simulink library "pelib"  (R2021a)
settings: Solver=VariableStepAuto  StartTime=0.0  StopTime=10.0  RelTol=1e-3
libraries: hdlBasic x7
settings Model: Creator=asc8  LastModifiedBy=asc8

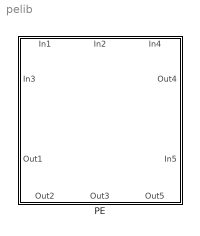
== system pelib ==
  PE : Subsystem
      settings: PortSchema="{\"entries\":[{\"content\":{\"sides\":[{\"content\":{\"connectorIds\":[\"In1\",\"Out5\"]},\"type\":\"ConnectorPlacement.EquallySpacedRectSide\",\"uuid\":\"f7e55443-70fb-4ed5-ab4f-147f7311106a\"},{\"content\":{\"connectorIds\":[\"Out1\",\"In5\"],\"side\":\"RIGHT\"},\"type\":\"ConnectorPlacement.EquallySpacedRectSide\",\"uuid\":\"6de0769a-4a22-4abb-b630-26d0c175204f\"},{\"content\":{\"connectorIds\":[\"In2\",\"In3\",\"In4\"],\"side\":\"TOP\"},\"type\":\"ConnectorPlacement.EquallySpacedRectSide\",\"uuid\":\"a041cc58-78e8-4444-b053-dd6f2c27badd\"},{\"content\":{\"connectorIds\":[\"Out2\",\"Out3\",\"Out4\"],\"side\":\"BOTTOM\"},\"type\":\"ConnectorPlacement.EquallySpacedRectSide\",\"uuid\":\"085ff6f5-8624-4aab-b622-9beedcd77ebd\"}]},\"type\":\"ConnectorPlacement.EquallySpacedConnector\",\"uuid\":\"928950cd-8b9e-4ebf-b8fd-b98c3e494fdc\"}],\"packageUris\":[\"http://schema.mathworks.com/mf0/Connector/R2020b\"],\"version\":\"1.0\"}"

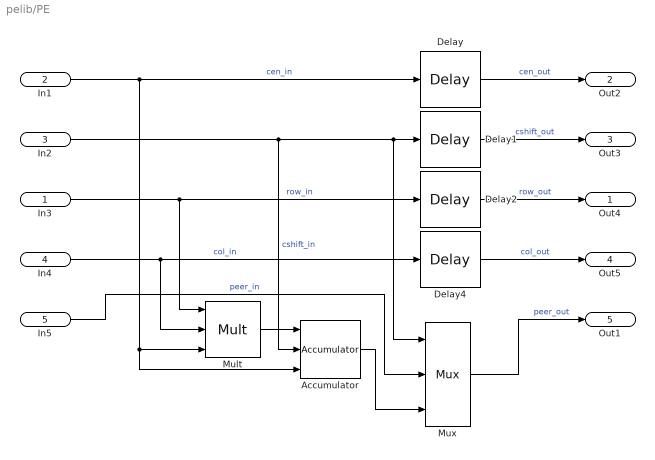
== system pelib/PE ==
  In3 : Inport
  In1 : Inport  Port=2
  In2 : Inport  Port=3
  In4 : Inport  Port=4
  In5 : Inport  Port=5
  Accumulator : hdlBasic/Accumulator  operation=Add  n_bits=16  overflow=Wrap  scale=1  rst=on  hasbypass=on  en=on  latency=1  msb_inp=100  msb=100  lsb=-100  use_behavioral_HDL=on  implementation=Fabric  XmcBlockStatus=1  maskContainerNames=group3  block_type=accum  block_config=sysgen:Accum_config
  Delay{,1..2,4} (4 alike) : hdlBasic/Delay  rst=off  en=off  latency=1  reg_retiming=off  XmcBlockStatus=1  maskContainerNames=group1  block_type=delay  block_config=sysgen:Delay_config
  Mult : hdlBasic/Mult  precision=User Defined  arith_type="Signed  (2's comp)"  n_bits=16  bin_pt=0  quantization=Truncate  overflow=Wrap  en=on  latency=2  use_behavioral_HDL=off  opt=Speed  use_embedded=on  optimum_pipeline=off  pipeline=on  use_rpm=on  placement_style=Triangular  XmcBlockStatus=1  maskContainerNames=group1  block_type=mult  block_config=sysgen:Mult_config
  Mux : hdlBasic/Mux  inputs=2  en=off  latency=0  precision=Full  arith_type=Unsigned  n_bits=16  bin_pt=14  quantization=Truncate  overflow=Wrap  XmcBlockStatus=1  maskContainerNames=tabcontainer1  block_type=mux  block_config=sysgen:Mux_config
  Out4 : Outport
  Out2 : Outport  Port=2
  Out3 : Outport  Port=3
  Out5 : Outport  Port=4
  Out1 : Outport  Port=5
  wires:
  In3/1 -> Mult/1, Delay2/1  "row_in"
  In4/1 -> Delay4/1, Mult/2  "col_in"
  In1/1 -> Mult/3, Accumulator/3, Delay/1  "cen_in"
  In2/1 -> Accumulator/2, Delay1/1, Mux/1  "cshift_in"
  Delay/1 -> Out2/1  "cen_out"
  Delay1/1 -> Out3/1  "cshift_out"
  Accumulator/1 -> Mux/3
  Mux/1 -> Out1/1  "peer_out"
  Delay2/1 -> Out4/1  "row_out"
  Delay4/1 -> Out5/1  "col_out"
  In5/1 -> Mux/2  "peer_in"
  Mult/1 -> Accumulator/1
